simulink model "uio"  (R2018a)
settings: Solver=VariableStepAuto  StartTime=0.0  StopTime=10.0  RelTol=1e-3
values from neighbouring files (symbols this model uses):
  T1 = 0.4    [SimulinkInit_linea_transmision.m]
  T2 = 1    [SimulinkInit_linea_transmision.m]
  T3 = 15    [SimulinkInit_linea_transmision.m]
  T4 = 2.5    [SimulinkInit_linea_transmision.m]
  T5 = 3.3    [SimulinkInit_linea_transmision.m]
undefined symbols (not defined in the file or in its folder): Bd, C10o, C11o, C12o, C1o, C2o, C3o, C4o, C5o, C6o, C7o, C8o, C9o, F1, F10, F11, F12, F2, F3, F4, F5, F6, F7, F8, F9, H1, H10, H11, H12, H2, H3, H4, H5, H6, H7, H8, H9, K10U, K11U, K12U, K1U, K2U, K3U, K4U, K5U, K6U, K7U, K8U, K9U, T10, T11, T12, T6, T7, T8, T9, tm
settings Model: Creator=MarioAndres  LastModifiedBy=MarioAndres

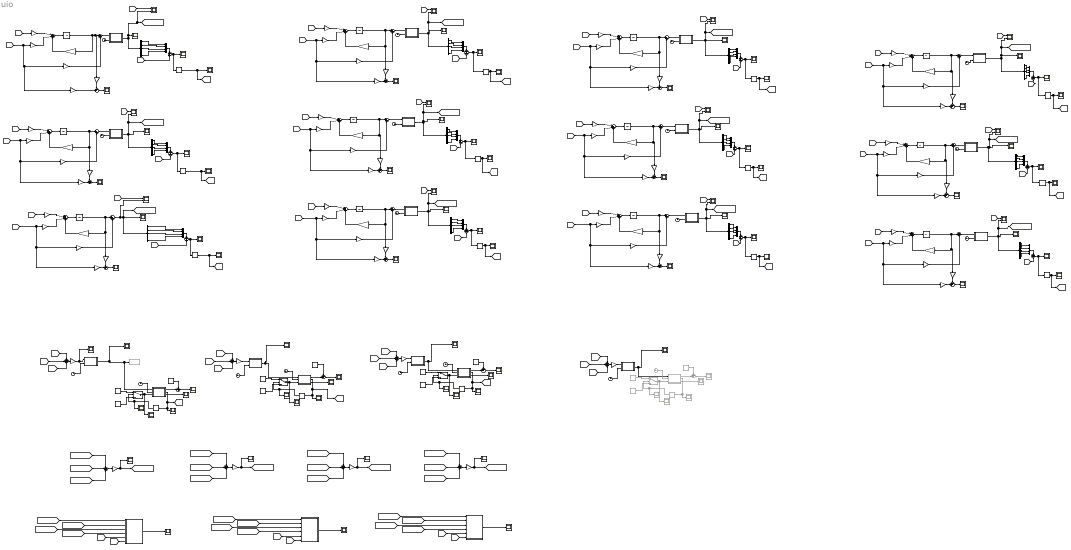
== system uio ==
  Clock{2..14,18..22} (18 alike) : Clock
  Clock15 : Clock  Commented=on
  Constant{4..6,8,10,24} (6 alike) : Constant
  Constant12 : Constant  Value=0
  Constant21 : Constant  Commented=on  Value=0
  Constant22 : Constant  Commented=on
  Constant23 : Constant  Value=0
  Constant7 : Constant  Value=0
  Constant9 : Constant  Commented=on
  Demux{1,4..14} (12 alike) : Demux  Outputs=5
  Derivative{,1,3,5..13} (12 alike) : Derivative  CoefficientInTFapproximation=0
  Gain{22..26,30..32} (8 alike) : Gain  Gain=1/3
  MATLAB Function : MATLAB Function  TreatAsAtomicUnit=on
  MATLAB Function10 : MATLAB Function  TreatAsAtomicUnit=on
  MATLAB Function11 : MATLAB Function  TreatAsAtomicUnit=on
  MATLAB Function12 : MATLAB Function  TreatAsAtomicUnit=on
  MATLAB Function13 : MATLAB Function  TreatAsAtomicUnit=on
  MATLAB Function14 : MATLAB Function  Commented=on  TreatAsAtomicUnit=on
  MATLAB Function23 : MATLAB Function  TreatAsAtomicUnit=on
  MATLAB Function24 : MATLAB Function  TreatAsAtomicUnit=on
  MATLAB Function25 : MATLAB Function  TreatAsAtomicUnit=on
  MATLAB Function26 : MATLAB Function  TreatAsAtomicUnit=on
  MATLAB Function27 : MATLAB Function  TreatAsAtomicUnit=on
  MATLAB Function28 : MATLAB Function  TreatAsAtomicUnit=on
  MATLAB Function29 : MATLAB Function  TreatAsAtomicUnit=on
  MATLAB Function30 : MATLAB Function  TreatAsAtomicUnit=on
  MATLAB Function31 : MATLAB Function  TreatAsAtomicUnit=on
  MATLAB Function32 : MATLAB Function  TreatAsAtomicUnit=on
  MATLAB Function33 : MATLAB Function  TreatAsAtomicUnit=on
  MATLAB Function34 : MATLAB Function  TreatAsAtomicUnit=on
  MATLAB Function36 : MATLAB Function  TreatAsAtomicUnit=on
  MATLAB Function38 : MATLAB Function  TreatAsAtomicUnit=on
  MATLAB Function39 : MATLAB Function  TreatAsAtomicUnit=on
  MATLAB Function9 : MATLAB Function  TreatAsAtomicUnit=on
  Memory : Memory
  Memory1 : Memory
  Memory2 : Memory
  Memory3 : Memory  Commented=on
  Mux{13,15..25} (12 alike) : Mux
  Scope{8..9,25,30..31,33..34,36,55..67,70..85,97,100..104,106,108..138} (75 alike) : Scope
  Scope{68..69,99,105,107} (5 alike) : Scope  Commented=on
  Scope{86..96,98} (12 alike) : Scope  NumInputPorts=2
  Sum{10,22,25,30,38..39,43,45,52,56,58,74} (12 alike) : Sum  Inputs=|++
  Sum{16,18,20,27..28,34,36,41,47,50,54,60} (12 alike) : Sum  Inputs=+-
  Sum{19,24,29,31..32,35,37,42,48,51,55,71} (12 alike) : Sum  Inputs=-+|
  Sum{21,23,26,33,40,44,46,49,53,57,59,76} (12 alike) : Sum  Inputs=|+++  SampleTime=tm
  Sum{61..63,67,69..70,72..73} (8 alike) : Sum  Inputs=+++
  Sum64 : Sum  Inputs=+-|
  Sum65 : Sum  Inputs=+-|
  Sum66 : Sum  Inputs=+-|
  Sum68 : Sum  Commented=on  Inputs=+-|
  Switch : Switch  Criteria=u2 > Threshold
  Switch1 : Switch  Criteria=u2 > Threshold
  Switch2 : Switch  Criteria=u2 > Threshold
  Switch3 : Switch  Commented=on  Criteria=u2 > Threshold
  To Workspace4 : ToWorkspace  Commented=on  VariableName=dr  SaveFormat=Structure With Time  SampleTime=-1
  Unit Delay{1..5,7..13} (12 alike) : UnitDelay  SampleTime=tm
  adis1 : Gain  Gain=F3  Multiplication=Matrix(K*u) (u vector)  SampleTime=tm
  adis11 : Gain  Gain=F1  Multiplication=Matrix(K*u) (u vector)  SampleTime=tm
  adis12 : Gain  Gain=F2  Multiplication=Matrix(K*u) (u vector)  SampleTime=tm
  adis13 : Gain  Gain=F11  Multiplication=Matrix(K*u) (u vector)  SampleTime=tm
  adis14 : Gain  Gain=F12  Multiplication=Matrix(K*u) (u vector)  SampleTime=tm
  adis2 : Gain  Gain=F4  Multiplication=Matrix(K*u) (u vector)  SampleTime=tm
  adis3 : Gain  Gain=F5  Multiplication=Matrix(K*u) (u vector)  SampleTime=tm
  adis4 : Gain  Gain=F6  Multiplication=Matrix(K*u) (u vector)  SampleTime=tm
  adis5 : Gain  Gain=F7  Multiplication=Matrix(K*u) (u vector)  SampleTime=tm
  adis6 : Gain  Gain=F8  Multiplication=Matrix(K*u) (u vector)  SampleTime=tm
  adis8 : Gain  Gain=F9  Multiplication=Matrix(K*u) (u vector)  SampleTime=tm
  adis9 : Gain  Gain=F10  Multiplication=Matrix(K*u) (u vector)  SampleTime=tm
  bdis1 : Gain  Gain=T3*Bd  Multiplication=Matrix(K*u) (u vector)  SampleTime=tm
  bdis10 : Gain  Gain=T2*Bd  Multiplication=Matrix(K*u) (u vector)  SampleTime=tm
  bdis11 : Gain  Gain=K2U  Multiplication=Matrix(K*u) (u vector)  SampleTime=tm
  bdis12 : Gain  Gain=H2  Multiplication=Matrix(K*u) (u vector)  SampleTime=tm
  bdis13 : Gain  Gain=eye(1)-C2o*H2  Multiplication=Matrix(K*u) (u vector)  SampleTime=tm
  bdis14 : Gain  Gain=eye(1)-C1o*H1  Multiplication=Matrix(K*u) (u vector)  SampleTime=tm
  bdis15 : Gain  Gain=C1o  Multiplication=Matrix(K*u) (u vector)  SampleTime=tm
  bdis16 : Gain  Gain=C2o  Multiplication=Matrix(K*u) (u vector)  SampleTime=tm
  bdis17 : Gain  Gain=T4*Bd  Multiplication=Matrix(K*u) (u vector)  SampleTime=tm
  bdis18 : Gain  Gain=K4U  Multiplication=Matrix(K*u) (u vector)  SampleTime=tm
  bdis19 : Gain  Gain=H4  Multiplication=Matrix(K*u) (u vector)  SampleTime=tm
  bdis2 : Gain  Gain=K3U  Multiplication=Matrix(K*u) (u vector)  SampleTime=tm
  bdis20 : Gain  Gain=eye(1)-C4o*H4  Multiplication=Matrix(K*u) (u vector)  SampleTime=tm
  bdis21 : Gain  Gain=C4o  Multiplication=Matrix(K*u) (u vector)  SampleTime=tm
  bdis22 : Gain  Gain=T5*Bd  Multiplication=Matrix(K*u) (u vector)  SampleTime=tm
  bdis23 : Gain  Gain=K5U  Multiplication=Matrix(K*u) (u vector)  SampleTime=tm
  bdis24 : Gain  Gain=H5  Multiplication=Matrix(K*u) (u vector)  SampleTime=tm
  bdis25 : Gain  Gain=eye(1)-C5o*H5  Multiplication=Matrix(K*u) (u vector)  SampleTime=tm
  bdis26 : Gain  Gain=C5o  Multiplication=Matrix(K*u) (u vector)  SampleTime=tm
  bdis27 : Gain  Gain=T6*Bd  Multiplication=Matrix(K*u) (u vector)  SampleTime=tm
  bdis28 : Gain  Gain=K6U  Multiplication=Matrix(K*u) (u vector)  SampleTime=tm
  bdis29 : Gain  Gain=H6  Multiplication=Matrix(K*u) (u vector)  SampleTime=tm
  bdis3 : Gain  Gain=H3  Multiplication=Matrix(K*u) (u vector)  SampleTime=tm
  bdis30 : Gain  Gain=eye(1)-C6o*H6  Multiplication=Matrix(K*u) (u vector)  SampleTime=tm
  bdis31 : Gain  Gain=C6o  Multiplication=Matrix(K*u) (u vector)  SampleTime=tm
  bdis32 : Gain  Gain=T7*Bd  Multiplication=Matrix(K*u) (u vector)  SampleTime=tm
  bdis33 : Gain  Gain=K7U  Multiplication=Matrix(K*u) (u vector)  SampleTime=tm
  bdis34 : Gain  Gain=H7  Multiplication=Matrix(K*u) (u vector)  SampleTime=tm
  bdis35 : Gain  Gain=eye(1)-C7o*H7  Multiplication=Matrix(K*u) (u vector)  SampleTime=tm
  bdis36 : Gain  Gain=C7o  Multiplication=Matrix(K*u) (u vector)  SampleTime=tm
  bdis37 : Gain  Gain=T8*Bd  Multiplication=Matrix(K*u) (u vector)  SampleTime=tm
  bdis38 : Gain  Gain=K8U  Multiplication=Matrix(K*u) (u vector)  SampleTime=tm
  bdis39 : Gain  Gain=H8  Multiplication=Matrix(K*u) (u vector)  SampleTime=tm
  bdis4 : Gain  Gain=eye(1)-C3o*H3  Multiplication=Matrix(K*u) (u vector)  SampleTime=tm
  bdis40 : Gain  Gain=eye(1)-C8o*H8  Multiplication=Matrix(K*u) (u vector)  SampleTime=tm
  bdis41 : Gain  Gain=C8o  Multiplication=Matrix(K*u) (u vector)  SampleTime=tm
  bdis42 : Gain  Gain=T9*Bd  Multiplication=Matrix(K*u) (u vector)  SampleTime=tm
  bdis43 : Gain  Gain=K9U  Multiplication=Matrix(K*u) (u vector)  SampleTime=tm
  bdis44 : Gain  Gain=H9  Multiplication=Matrix(K*u) (u vector)  SampleTime=tm
  bdis45 : Gain  Gain=eye(1)-C9o*H9  Multiplication=Matrix(K*u) (u vector)  SampleTime=tm
  bdis46 : Gain  Gain=C9o  Multiplication=Matrix(K*u) (u vector)  SampleTime=tm
  bdis47 : Gain  Gain=T10*Bd  Multiplication=Matrix(K*u) (u vector)  SampleTime=tm
  bdis48 : Gain  Gain=K10U  Multiplication=Matrix(K*u) (u vector)  SampleTime=tm
  bdis49 : Gain  Gain=H10  Multiplication=Matrix(K*u) (u vector)  SampleTime=tm
  bdis50 : Gain  Gain=eye(1)-C10o*H10  Multiplication=Matrix(K*u) (u vector)  SampleTime=tm
  bdis51 : Gain  Gain=C10o  Multiplication=Matrix(K*u) (u vector)  SampleTime=tm
  bdis52 : Gain  Gain=T11*Bd  Multiplication=Matrix(K*u) (u vector)  SampleTime=tm
  bdis53 : Gain  Gain=K11U  Multiplication=Matrix(K*u) (u vector)  SampleTime=tm
  bdis54 : Gain  Gain=H11  Multiplication=Matrix(K*u) (u vector)  SampleTime=tm
  bdis55 : Gain  Gain=eye(1)-C11o*H11  Multiplication=Matrix(K*u) (u vector)  SampleTime=tm
  bdis56 : Gain  Gain=C11o  Multiplication=Matrix(K*u) (u vector)  SampleTime=tm
  bdis57 : Gain  Gain=T12*Bd  Multiplication=Matrix(K*u) (u vector)  SampleTime=tm
  bdis58 : Gain  Gain=K12U  Multiplication=Matrix(K*u) (u vector)  SampleTime=tm
  bdis59 : Gain  Gain=H12  Multiplication=Matrix(K*u) (u vector)  SampleTime=tm
  bdis6 : Gain  Gain=C3o  Multiplication=Matrix(K*u) (u vector)  SampleTime=tm
  bdis60 : Gain  Gain=eye(1)-C12o*H12  Multiplication=Matrix(K*u) (u vector)  SampleTime=tm
  bdis61 : Gain  Gain=C12o  Multiplication=Matrix(K*u) (u vector)  SampleTime=tm
  bdis7 : Gain  Gain=T1*Bd  Multiplication=Matrix(K*u) (u vector)  SampleTime=tm
  bdis8 : Gain  Gain=K1U  Multiplication=Matrix(K*u) (u vector)  SampleTime=tm
  bdis9 : Gain  Gain=H1  Multiplication=Matrix(K*u) (u vector)  SampleTime=tm
  wires:
  Sum40/1 -> Unit Delay8/1
  bdis33/1 -> Sum46/2
  Unit Delay4/1 -> bdis31/1, adis4/1, Sum30/1
  Sum33/1 -> Unit Delay4/1
  Demux12/3 -> Mux20/3
  Clock3/1 -> MATLAB Function/2(t)
  [u_fs] -> bdis37/1
  Demux7/3 -> Mux18/3
  Constant9/1 -> Sum68/1
  bdis8/1 -> Sum21/2
  bdis45/1 -> Sum42/2
  Demux5/2 -> Mux16/2
  [I3] -> bdis25/1, bdis24/1, bdis23/1
  Sum55/1 -> Scope77/1
  bdis28/1 -> Sum33/2
  bdis25/1 -> Sum24/2
  [u_fs] -> bdis57/1
  [druo8] -> Sum63/2
  Sum30/1 -> MATLAB Function27/1(u)
  Derivative/1 -> [druo1], Scope106/1
  bdis30/1 -> Sum29/2
  Sum57/1 -> Unit Delay13/1
  Derivative1/1 -> [druo2], Scope111/1
  Demux8/2 -> Mux19/2
  Demux1/1 -> Mux13/1
  [rol] -> MATLAB Function39/6(rol)
  Gain23/1 -> MATLAB Function13/1(u)
  Demux8/3 -> Mux19/3
  Gain25/1 -> Scope135/1, [x_hat_uio4]
  Demux12/2 -> Mux20/2
  Sum64/1 -> Scope120/1
  Sum74/1 -> MATLAB Function25/1(u)
  bdis43/1 -> Sum44/2
  Constant4/1 -> Sum64/1
  bdis19/1 -> Sum74/2
  [x_hat_uio41] -> Sum73/1
  bdis51/1 -> Sum48/1
  Demux1/3 -> Mux13/3
  Sum22/1 -> MATLAB Function24/1(u)
  Demux11/1 -> Mux25/1
  Constant23/1 -> Switch/1
  Mux15/1 -> Sum47/1
  [druo7] -> Sum63/1
  Gain32/1 -> Scope114/1, [x_hat_uio2]
  [x_hat_uio32] -> Sum72/2
  Memory1/1 -> Scope129/1, Switch1/2
  MATLAB Function13/1(y) -> MATLAB Function11/1(dr), Scope110/1
  adis9/1 -> Sum59/3
  MATLAB Function11/1(r) -> Sum65/2
  Switch1/1 -> Scope127/1, MATLAB Function11/3(ban)
  Sum65/1 -> Scope125/1
  [x_hat_uio1] -> MATLAB Function39/1(x_hat1)
  [I2] -> bdis55/1, bdis54/1, bdis53/1
  Sum60/1 -> Derivative3/1, Scope64/1
  Clock10/1 -> MATLAB Function30/2(t)
  [y_ma] -> Sum27/2
  MATLAB Function28/1(y) -> Demux10/1, [x_hat_uio31], Scope92/2, Scope36/1
  Demux11/2 -> Mux25/2
  [y_ma] -> Sum47/2
  Demux14/3 -> Mux24/3
  Mux19/1 -> Sum18/1
  Derivative8/1 -> [druo7], Scope119/1
  [x_hat_uio21] -> Sum70/1
  MATLAB Function30/1(y) -> Demux14/1, [x_hat_uio33], Scope94/2, Scope75/1
  Mux25/1 -> Sum50/1
  adis6/1 -> Sum40/3
  Sum21/1 -> Unit Delay7/1
  Gain26/1 -> MATLAB Function10/1(u)
  [y_ma] -> Sum16/2
  Mux20/1 -> Sum54/1
  Sum25/1 -> MATLAB Function26/1(u)
  bdis10/1 -> Sum23/1
  Mux23/1 -> Sum34/1
  Derivative13/1 -> [druo9], Scope101/1
  [y_ma] -> Sum18/2
  [y_ma] -> Scope93/1
  Sum41/1 -> Derivative13/1, Scope25/1
  Clock5/1 -> MATLAB Function25/2(t)
  [druo1] -> Sum61/1
  Clock20/1 -> MATLAB Function36/2(t)
  Sum54/1 -> Derivative12/1, Scope76/1
  Demux13/1 -> Mux15/1
  Gain30/1 -> MATLAB Function12/1(u)
  MATLAB Function36/3(o) -> Scope123/1
  [u_fs] -> bdis17/1
  Clock22/1 -> MATLAB Function23/2(t)
  [x_hat_uio3] -> MATLAB Function34/3(x_hat3)
  Switch/1 -> Scope122/1, MATLAB Function36/3(ban)
  Sum18/1 -> Derivative5/1, Scope71/1
  [y_ma] -> Scope86/1
  [y_ma] -> Scope95/1
  Sum67/1 -> Gain30/1
  Sum42/1 -> Scope31/1
  [u_fs] -> bdis32/1
  Sum48/1 -> Scope83/1
  MATLAB Function23/1(r) -> Sum66/2
  Sum46/1 -> Unit Delay5/1
  bdis29/1 -> Sum30/2
  MATLAB Function24/1(y) -> Demux6/1, [x_hat_uio12], Scope87/2, Scope58/1
  Derivative12/1 -> [druo12], Scope104/1
  Memory/1 -> Scope124/1, Switch/2
  Sum39/1 -> MATLAB Function29/1(u)
  Sum53/1 -> Unit Delay12/1
  MATLAB Function32/1(y) -> Demux12/1, [x_hat_uio43], Scope98/2, Scope85/1
  MATLAB Function38/1(v1) -> Scope109/1
  Demux10/2 -> Mux23/2
  Clock21/1 -> MATLAB Function11/2(t)
  Derivative6/1 -> [druo5], Scope116/1
  MATLAB Function10/1(y) -> MATLAB Function23/1(dr), Scope112/1
  Demux5/3 -> Mux16/3
  bdis52/1 -> Sum53/1
  Constant5/1 -> Switch1/3
  Mux16/1 -> Sum16/1
  Sum16/1 -> Derivative/1, Scope59/1
  Derivative11/1 -> [druo11], Scope103/1
  [y_ma] -> Scope91/1
  Memory2/1 -> Scope134/1, Switch2/2
  Derivative7/1 -> [druo6], Scope117/1
  [x_hat_uio2] -> MATLAB Function39/2(x_hat2)
  [x_hat_uio42] -> Sum73/2
  Sum71/1 -> Scope67/1
  MATLAB Function39/1(v1) -> Scope137/1
  [y_ma] -> Scope96/1
  [rol] -> MATLAB Function38/6(rol)
  bdis42/1 -> Sum44/1
  bdis17/1 -> Sum76/1
  [ruo1] -> MATLAB Function38/5(ruo1)
  MATLAB Function33/1(y) -> Demux11/1, [x_hat_uio42], Scope96/2, Scope78/1
  Sum68/1 -> Scope68/1
  [druo10] -> Sum67/1
  Sum61/1 -> Gain22/1
  Unit Delay1/1 -> bdis6/1, adis1/1, Sum38/1
  MATLAB Function23/2(c) -> [ruo3], Scope131/1, Memory2/1
  Gain24/1 -> Scope118/1, [x_hat_uio3]
  Demux5/1 -> Mux16/1
  MATLAB Function34/1(v1) -> Scope136/1
  Sum72/1 -> Gain24/1
  bdis20/1 -> Sum19/2
  [druo5] -> Sum62/2
  Demux6/1 -> Mux17/1
  Gain31/1 -> Scope138/1, [x_hat_uio1]
  adis14/1 -> Sum57/3
  Sum35/1 -> Scope73/1
  bdis16/1 -> Sum32/1
  [x_hat_uio4] -> MATLAB Function34/4(x_hat4)
  bdis1/1 -> Sum49/1
  [druo11] -> Sum67/2
  MATLAB Function23/3(o) -> Scope133/1
  Gain22/1 -> Scope30/1, MATLAB Function9/1(u)
  [x_hat_uio11] -> Sum69/1
  [druo12] -> Sum67/3
  bdis56/1 -> Sum51/1
  [x_hat_uio31] -> Sum72/1
  bdis47/1 -> Sum59/1
  Constant22/1 -> Switch3/3
  Sum29/1 -> Scope9/1
  Constant24/1 -> Switch/3
  [V_vsi] -> bdis45/1, bdis44/1, bdis43/1
  [x_hat_uio1] -> MATLAB Function34/1(x_hat1)
  Demux10/5 -> Mux23/4
  MATLAB Function14/1(r) -> Sum68/2
  [x_hat_uio33] -> Sum72/3
  Derivative5/1 -> [druo4], Scope115/1
  Sum31/1 -> Scope65/1
  Memory3/1 -> Scope107/1, Switch3/2
  Clock2/1 -> MATLAB Function9/2(t)
  [x_hat_uio1] -> MATLAB Function38/1(x_hat1)
  [y_ma] -> Sum41/2
  bdis11/1 -> Sum23/2
  MATLAB Function14/2(c) -> Scope69/1, Memory3/1
  Sum66/1 -> Scope130/1
  Sum43/1 -> MATLAB Function30/1(u)
  Demux7/1 -> Mux18/1
  [y_ma] -> Sum50/2
  Sum73/1 -> Gain25/1
  Clock6/1 -> MATLAB Function26/2(t)
  [x_hat_uio2] -> MATLAB Function38/2(x_hat2)
  [x_hat_uio13] -> Sum69/3
  Sum56/1 -> MATLAB Function32/1(u)
  Demux7/2 -> Mux18/2
  Demux13/2 -> Mux15/2
  MATLAB Function14/3(o) -> Scope105/1
  Sum62/1 -> Gain23/1
  [x_hat_uio4] -> MATLAB Function39/4(x_hat4)
  bdis34/1 -> Sum45/2
  Clock14/1 -> MATLAB Function12/2(t)
  [I2] -> bdis40/1, bdis39/1, bdis38/1
  MATLAB Function12/1(y) -> MATLAB Function14/1(dr), Scope56/1
  Sum70/1 -> Gain32/1
  bdis7/1 -> Sum21/1
  Constant10/1 -> Sum65/1
  Demux6/5 -> Mux17/4
  MATLAB Function26/1(y) -> Scope57/1, [x_hat_uio22], Scope90/2, Demux1/1
  [x_hat_uio3] -> MATLAB Function38/3(x_hat3)
  adis13/1 -> Sum53/3
  Demux9/1 -> Mux22/1
  [x_hat_uio4] -> MATLAB Function38/4(x_hat4)
  [x_hat_uio2] -> MATLAB Function34/2(x_hat2)
  Clock15/1 -> MATLAB Function14/2(t)
  Constant7/1 -> Switch2/1
  Clock7/1 -> MATLAB Function27/2(t)
  Switch2/1 -> Scope132/1, MATLAB Function23/3(ban)
  Constant8/1 -> Switch2/3
  Clock19/1 -> MATLAB Function10/2(t)
  [x_hat_uio12] -> Sum69/2
  Sum69/1 -> Gain31/1
  Unit Delay3/1 -> bdis26/1, adis3/1, Sum25/1
  MATLAB Function11/3(o) -> Scope128/1
  bdis27/1 -> Sum33/1
  Demux13/3 -> Mux15/3
  Sum26/1 -> Unit Delay3/1
  Sum44/1 -> Unit Delay9/1
  [V_vsi] -> bdis4/1, bdis3/1, bdis2/1
  MATLAB Function/1(y) -> Scope61/1, [x_hat_uio11], Scope86/2, Demux5/1
  Demux10/1 -> Mux23/1
  [y_ma] -> Sum54/2
  [x_hat_uio23] -> Sum70/3
  [u_fs] -> bdis47/1
  Clock11/1 -> MATLAB Function31/2(t)
  bdis18/1 -> Sum76/2
  Sum52/1 -> MATLAB Function33/1(u)
  [x_hat_uio22] -> Sum70/2
  Demux10/3 -> Mux23/3
  Mux18/1 -> Sum60/1
  [y_ma] -> Scope92/1
  Sum36/1 -> Derivative9/1, Scope34/1
  bdis48/1 -> Sum59/2
  Clock18/1 -> MATLAB Function13/2(t)
  Unit Delay8/1 -> bdis41/1, adis6/1, Sum39/1
  Sum28/1 -> Derivative7/1, Scope8/1
  [I1] -> bdis20/1, bdis19/1, bdis18/1
  Demux8/5 -> Mux19/4
  Demux6/3 -> Mux17/3
  [druo6] -> Sum62/3
  bdis58/1 -> Sum57/2
  bdis55/1 -> Sum51/2
  Clock8/1 -> MATLAB Function28/2(t)
  [y_ma] -> Scope90/1
  Derivative3/1 -> [druo3], Scope113/1
  Unit Delay2/1 -> bdis21/1, adis2/1, Sum74/1
  [y_ma] -> Sum34/2
  Sum47/1 -> Derivative10/1, Scope82/1
  Derivative9/1 -> [druo8], Scope100/1
  Demux11/5 -> Mux25/4
  bdis61/1 -> Sum55/1
  MATLAB Function25/1(y) -> Scope70/1, [x_hat_uio21], Scope89/2, Demux8/1
  MATLAB Function27/1(y) -> Demux4/1, [x_hat_uio23], Scope91/2, Scope97/1
  bdis40/1 -> Sum37/2
  bdis60/1 -> Sum55/2
  bdis38/1 -> Sum40/2
  bdis35/1 -> Sum35/2
  Demux8/1 -> Mux19/1
  [u_fs] -> bdis7/1
  [y_ma] -> Scope94/1
  [y_ma] -> Sum20/2
  bdis39/1 -> Sum39/2
  [I2] -> bdis14/1, bdis9/1, bdis8/1
  MATLAB Function36/1(r) -> Sum64/2
  Sum63/1 -> Gain26/1
  bdis13/1 -> Sum32/2
  Demux1/5 -> Mux13/4
  bdis44/1 -> Sum43/2
  MATLAB Function36/2(c) -> [ruo1], Scope121/1, Memory/1
  [y_ma] -> Scope87/1
  adis1/1 -> Sum49/3
  bdis50/1 -> Sum48/2
  [y_ma] -> Scope98/1
  Unit Delay5/1 -> bdis36/1, adis5/1, Sum45/1
  bdis23/1 -> Sum26/2
  Demux1/2 -> Mux13/2
  Demux12/1 -> Mux20/1
  bdis53/1 -> Sum53/2
  [y_ma] -> Sum60/2
  Derivative10/1 -> [druo10], Scope102/1
  adis2/1 -> Sum76/3
  Switch3/1 -> Scope99/1, MATLAB Function14/3(ban)
  bdis41/1 -> Sum37/1
  Demux9/5 -> Mux22/4
  adis8/1 -> Sum44/3
  Sum19/1 -> Scope72/1
  Demux4/2 -> Mux21/2
  Sum27/1 -> Derivative1/1, Scope60/1
  bdis46/1 -> Sum42/1
  [u_fs] -> bdis27/1
  Unit Delay9/1 -> bdis46/1, adis8/1, Sum43/1
  bdis22/1 -> Sum26/1
  bdis32/1 -> Sum46/1
  [x_hat_uio43] -> Sum73/3
  bdis2/1 -> Sum49/2
  Constant21/1 -> Switch3/1
  adis4/1 -> Sum33/3
  [ruo3] -> MATLAB Function39/5(ruo1)
  MATLAB Function9/1(y) -> Scope108/1, MATLAB Function36/1(dr), To Workspace4/1
  Mux13/1 -> Sum20/1
  [y_ma] -> Scope89/1
  Sum51/1 -> Scope84/1
  Demux7/5 -> Mux18/4
  [I3] -> bdis13/1, bdis12/1, bdis11/1
  Mux22/1 -> Sum36/1
  bdis4/1 -> Sum71/2
  [u_fs] -> bdis42/1
  bdis14/1 -> Sum31/2
  MATLAB Function11/2(c) -> [ruo2], Scope126/1, Memory1/1
  bdis12/1 -> Sum22/2
  Sum20/1 -> Derivative6/1, Scope63/1
  bdis57/1 -> Sum57/1
  Mux21/1 -> Sum28/1
  [y_ma] -> Sum36/2
  [druo9] -> Sum63/3
  Sum24/1 -> Scope79/1
  bdis15/1 -> Sum31/1
  [x_hat_uio3] -> MATLAB Function39/3(x_hat3)
  [u_fs] -> bdis10/1
  bdis49/1 -> Sum58/2
  Unit Delay7/1 -> adis11/1, bdis15/1, Sum10/1
  Demux14/1 -> Mux24/1
  Sum10/1 -> MATLAB Function/1(u)
  [druo4] -> Sum62/1
  Sum59/1 -> Unit Delay11/1
  bdis36/1 -> Sum35/1
  [ruo2] -> MATLAB Function34/5(ruo1)
  adis5/1 -> Sum46/3
  Demux14/5 -> Mux24/4
  Demux4/3 -> Mux21/3
  Unit Delay11/1 -> bdis51/1, adis9/1, Sum58/1
  [u_fs] -> bdis1/1
  Clock4/1 -> MATLAB Function24/2(t)
  bdis26/1 -> Sum24/1
  Demux14/2 -> Mux24/2
  [I1] -> bdis50/1, bdis49/1, bdis48/1
  bdis37/1 -> Sum40/1
  Demux9/3 -> Mux22/3
  bdis54/1 -> Sum52/2
  Sum32/1 -> Scope66/1
  Demux6/2 -> Mux17/2
  Sum76/1 -> Unit Delay2/1
  Clock13/1 -> MATLAB Function33/2(t)
  Sum49/1 -> Unit Delay1/1
  Demux5/5 -> Mux16/4
  Constant6/1 -> Sum66/1
  [druo2] -> Sum61/2
  Demux4/5 -> Mux21/4
  Sum58/1 -> MATLAB Function31/1(u)
  Clock12/1 -> MATLAB Function32/2(t)
  [druo3] -> Sum61/3
  bdis24/1 -> Sum25/2
  adis3/1 -> Sum26/3
  bdis3/1 -> Sum38/2
  Sum50/1 -> Derivative11/1, Scope80/1
  MATLAB Function31/1(y) -> [x_hat_uio41], Scope95/2, Scope81/1, Demux13/1
  Sum34/1 -> Derivative8/1, Scope55/1
  [I1] -> bdis35/1, bdis34/1, bdis33/1
  Demux4/1 -> Mux21/1
  Sum45/1 -> MATLAB Function28/1(u)
  bdis31/1 -> Sum29/1
  adis11/1 -> Sum21/3
  Unit Delay12/1 -> bdis56/1, adis13/1, Sum52/1
  [I3] -> bdis60/1, bdis59/1, bdis58/1
  Demux11/3 -> Mux25/3
  Demux13/5 -> Mux15/4
  [y_ma] -> Sum28/2
  Unit Delay10/1 -> bdis16/1, adis12/1, Sum22/1
  Clock9/1 -> MATLAB Function29/2(t)
  bdis6/1 -> Sum71/1
  [y_ma] -> Scope88/1
  Mux24/1 -> Sum41/1
  Unit Delay13/1 -> bdis61/1, adis14/1, Sum56/1
  Demux12/5 -> Mux20/4
  Sum23/1 -> Unit Delay10/1
  [u_fs] -> bdis52/1
  [rol] -> MATLAB Function34/6(rol)
  bdis21/1 -> Sum19/1
  bdis59/1 -> Sum56/2
  MATLAB Function29/1(y) -> Demux9/1, [x_hat_uio32], Scope93/2, Scope33/1
  Sum37/1 -> Scope74/1
  Sum38/1 -> [x_hat_uio13], Demux7/1, Scope62/1, Scope88/2
  Mux17/1 -> Sum27/1
  adis12/1 -> Sum23/3
  Constant12/1 -> Switch1/1
  [V_vsi] -> bdis30/1, bdis29/1, bdis28/1
  [u_fs] -> bdis22/1
  Demux9/2 -> Mux22/2
  bdis9/1 -> Sum10/2

== matlab function uio/MATLAB Function ==
  data: u input; y output; t input
function y = fcn(u,t)
y1=u(1);
y2=u(2);
if t<=0.33
    y3=u(3)*0.69;%*0.52;
else
    y3=u(3)*0.52;
end
y4=u(4);
y5=u(5);
y = [y1 y2 y3 y4 y5];

== matlab function uio/MATLAB Function9 ==
  data: u input; y output; t input
function y = fcn(u,t)
y=[0 0 0 0];
if t<=0.04
    y =[0 0 0 0];
else
    y1=u(1)*(10^5)/(10^16);
    y2=u(2)*(10^5)/(10^16);
    y3=u(3)*(10^5)/(10^16);
    y4=u(4)*(10^5)/(10^16);
    y=[y1 y2 y3 y4];
end

== matlab function uio/MATLAB Function14 ==
  data: dr input; r output; t input; ban input; c output; o output
function [r,c,o]   = fcn(dr,t,ban)

if t<=0.33
    th=2e4;
    %     v=2;
else
    th=1e4;
    %     v=3;
end

% r=0;
% c=1;

if ban==1
    r=1;
    c=0;
    if abs(dr(3))>th
        c=1;
        r=0;
    end
else
    r=0;
    c=1;
    if abs(dr(3))>th %%&& ban==0
        c=0;
        r=1;
    end
end

% ra=r;
% a=0;
o=abs(dr(4));

== matlab function uio/MATLAB Function13 ==
  data: u input; y output; t input
function y = fcn(u,t)
y=[0 0 0 0];
if t<=0.1
    y =[0 0 0 0];
else
    y1=u(1)*(10^5)/(10^16);
    y2=u(2)*(10^5)/(10^16);
    y3=u(3)*(10^5)/(10^16);
    y4=u(4)*(10^5)/(10^16);
    y=[y1 y2 y3 y4];
end

== matlab function uio/MATLAB Function24 ==
  data: u input; y output; t input
function y = fcn(u,t)
y1=u(1);
y2=u(2);
if t>0.33
    y2=u(2)*1.31;%*0.52;
    y5=u(5)*1.55;
else
    y2=u(2);
    
    y5=u(5)*1.39;
    
end
y3=u(3);
y4=u(4);


y = [y1 y2 y3 y4 y5];

== matlab function uio/MATLAB Function25 ==
  data: u input; y output; t input
function y = fcn(u,t)
y1=u(1);
y2=u(2);
if t>0.33
    y3=u(3)*0.54+5;
    y5=u(5)*1.15;
else
    y3=u(3)*0.7;
    
    y5=u(5);
    
end

y4=u(4);


y = [y1 y2 y3 y4 y5];

== matlab function uio/MATLAB Function26 ==
  data: u input; y output; t input
function y = fcn(u,t)
y1=u(1);
y2=u(2);
if t>0.33
    y2=u(2)*1.32;
    y5=u(5)*1.52;
else
    y2=u(2);
    y5=u(5)*1.4;
      
end
y3=u(3);
y4=u(4);



y = [y1 y2 y3 y4 y5];

== matlab function uio/MATLAB Function27 ==
  data: u input; y output; t input
function y = fcn(u,t)
y1=u(1);
y2=u(2);
% if t>0.33
%     y2=u(2)*1.32;
%     y5=u(5)*1.52;
% else
%     y2=u(2);
%     y5=u(5)*1.4;
      
% end
y3=u(3);
y4=u(4);
y5=u(5);



y = [y1 y2 y3 y4 y5];

== matlab function uio/MATLAB Function28 ==
  data: u input; y output; t input
function y = fcn(u,t)
y1=u(1);
y2=u(2);
if t>0.33
    y3=u(3)*0.54+5;
    y5=u(5)*1.14;
else
    y3=u(3)*0.7;
    y5=u(5);
      
end
% y3=u(3);
y4=u(4);



y = [y1 y2 y3 y4 y5];

== matlab function uio/MATLAB Function29 ==
  data: u input; y output; t input
function y = fcn(u,t)
y1=u(1);
y2=u(2);
if t>0.33
    y3=u(3)*0.54;
%     y5=u(5)*1.14;
else
    y3=u(3)*0.7;
%     y5=u(5);
      
end
% y3=u(3);
y4=u(4);
y5=u(5);



y = [y1 y2 y3 y4 y5];

== matlab function uio/MATLAB Function30 ==
  data: u input; y output; t input
function y = fcn(u,t)
y1=u(1);
y2=u(2);
% if t>0.33
%     y3=u(3)*0.54;
% %     y5=u(5)*1.14;
% else
%     y3=u(3)*0.7;
% %     y5=u(5);
%       
% end
y3=u(3);
y4=u(4);
y5=u(5);



y = [y1 y2 y3 y4 y5];

== matlab function uio/MATLAB Function31 ==
  data: u input; y output; t input
function y = fcn(u,t)
y1=u(1);
y2=u(2);
if t>0.33
    y3=u(3)*0.54;
    y5=u(5)*1.13;
else
    y3=u(3)*0.7;
    y5=u(5);
      
end
% y3=u(3);
y4=u(4);
% y5=u(5);



y = [y1 y2 y3 y4 y5];

== matlab function uio/MATLAB Function32 ==
  data: u input; y output; t input
function y = fcn(u,t)
y1=u(1); %-5  +5

if t>0.33
    y2=u(2)*1.27;
    
    y5=u(5)*1.47;
else
    y2=u(2);
    
    y5=u(5)*1.34;
    
end
y3=u(3);
y4=u(4);
% y5=u(5);



y = [y1 y2 y3 y4 y5];

== matlab function uio/MATLAB Function33 ==
  data: u input; y output; t input
function y = fcn(u,t)
y1=u(1)-10;
y2=u(2);
if t>0.33
    y3=u(3)*0.54;
%     y5=u(5)*1.14;
else
    y3=u(3)*0.7;
%     y5=u(5);
      
end
% y3=u(3);
y4=u(4);
y5=u(5);



y = [y1 y2 y3 y4 y5];

== matlab function uio/MATLAB Function12 ==
  data: u input; y output; t input
function y = fcn(u,t)
y=[0 0 0 0];
if t<=0.3
    y =[0 0 0 0];
else
    y1=u(1)*(10^5)/(10^16);
    y2=u(2)*(10^5)/(10^16);
    y3=u(3)*(10^5)/(10^16);
    y4=u(4)*(10^5)/(10^16);
    y=[y1 y2 y3 y4];
end

== matlab function uio/MATLAB Function34 ==
  data: x_hat1 input; v1 output; x_hat2 input; x_hat3 input; x_hat4 input; ruo1 input; rol input
function v1 = fcn(x_hat1,x_hat2,x_hat3,x_hat4,ruo1,rol)

% yol=[u1 ; u2];
% ym=[ym1 ; ym2];
 C1=[0     1     0  0   0];
 v11=C1*(x_hat2'-x_hat1')*ruo1*rol;
 v12=C1*(x_hat2'-x_hat3')*ruo1*rol;
 v13=C1*(x_hat2'-x_hat4')*ruo1*rol;
 
 v1=(v11+v12+v13)/3;

== matlab function uio/MATLAB Function38 ==
  data: x_hat1 input; v1 output; x_hat2 input; x_hat3 input; x_hat4 input; ruo1 input; rol input
function v1 = fcn(x_hat1,x_hat2,x_hat3,x_hat4,ruo1,rol)

% yol=[u1 ; u2];
% ym=[ym1 ; ym2];
 C1=[1     0     0  0   0];
 v11=C1*(x_hat1'-x_hat2')*ruo1*rol;
 v12=C1*(x_hat1'-x_hat3')*ruo1*rol;
 v13=C1*(x_hat1'-x_hat4')*ruo1*rol;
 
 v1=(v11+v12+v13)/3;

== matlab function uio/MATLAB Function10 ==
  data: u input; y output; t input
function y = fcn(u,t)
y=[0 0 0 0];
if t<=0.3
    y =[0 0 0 0];
else
    y1=u(1)*(10^5)/(10^16);
    y2=u(2)*(10^5)/(10^16);
    y3=u(3)*(10^5)/(10^16);
    y4=u(4)*(10^5)/(10^16);
    y=[y1 y2 y3 y4];
end

== matlab function uio/MATLAB Function36 ==
  data: dr input; r output; t input; ban input; c output; o output
function [r,c,o]   = fcn(dr,t,ban)

if t<=0.33
    th=1.5e4;
    %     v=2;
elseif t<=0.55
    th=2e4;
    %     v=3;
else
    th=3e3;
end

% r=0;
% c=1;

if ban==1
    r=1;
    c=0;
    if abs(dr(1))>th
        c=1;
        r=0;
    end
else
    r=0;
    c=1;
    if abs(dr(1))>th %%&& ban==0
        c=0;
        r=1;
    end
end

% ra=r;
% a=0;
o=abs(dr(1));

== matlab function uio/MATLAB Function39 ==
  data: x_hat1 input; v1 output; x_hat2 input; x_hat3 input; x_hat4 input; ruo1 input; rol input
function v1 = fcn(x_hat1,x_hat2,x_hat3,x_hat4,ruo1,rol)

% yol=[u1 ; u2];
% ym=[ym1 ; ym2];
 C1=[0     0     1  0   0];
 v11=C1*(x_hat3'-x_hat1')*ruo1*rol;
 v12=C1*(x_hat3'-x_hat2')*ruo1*rol;
 v13=C1*(x_hat3'-x_hat4')*ruo1*rol;
 
 v1=(v11+v12+v13)/3;

== matlab function uio/MATLAB Function11 ==
  data: dr input; r output; t input; ban input; c output; o output
function [r,c,o]   = fcn(dr,t,ban)

if t<=0.33
    th=1e4;
    %     v=2;
elseif t<=0.5
    th=1e4;
    %     v=3;
elseif t>0.5 && t<=1
    th=3500;
else
    th=3000;
end

% r=0;
% c=1;

if ban==1
    r=1;
    c=0;
    if abs(dr(2))>th
        c=1;
        r=0;
    end
else
    r=0;
    c=1;
    if abs(dr(2))>th %%&& ban==0
        c=0;
        r=1;
    end
end

% ra=r;
% a=0;
o=abs(dr(2));

== matlab function uio/MATLAB Function23 ==
  data: dr input; r output; t input; ban input; c output; o output
function [r,c,o]   = fcn(dr,t,ban)

if t<=0.52
    th=2e4;
    %     v=2;
else
    th=0.7e4;%1e4;
    %     v=3;
end

% r=0;
% c=1;

if ban==1
    r=1;
    c=0;
    if abs(dr(3))>th
        c=1;
        r=0;
    end
else
    r=0;
    c=1;
    if abs(dr(3))>th %%&& ban==0
        c=0;
        r=1;
    end
end

% ra=r;
% a=0;
o=abs(dr(3));
